simulink model "CACC_system_struct"  (Simulink 8.2)
settings: Solver=ode1  SolverMode=SingleTasking  StartTime=0.0  StopTime=inf  FixedStep=0.01  RelTol=1e-3
PreLoadFcn:
  | numd_dvsp = [0.3579 0 -0.3579];
  | dend_dvsp = [1 -1.846 0.8535];
  | simpleacc_param
PostLoadFcn:
  | , if any(exist('dsrtsu_mdlpostloadfcn', 'file') == [2, 3, 6]), try dsrtsu_mdlpostloadfcn('Execute', bdroot); catch fprintf('Error in PostLoadFcn (dsrtsu_mdlpostloadfcn) for model "%s":\n %s\n', bdroot, lasterr); end, end,
undefined symbols (not defined in the file or in its folder): command_mode, max_accel_m_s2, override_enabled, speed_command_m_s, wrench_effort_command
libraries: carma_platform x3, dsrc_transmitter x2, rtitttasklib x2, lightbar x2, srx_platform x1
(part 1 of 4)
CloseFcn:
  | rtwprivate ssgencode ModelCloseRequest Y50_MABX
settings Model: DSRTSU_INTERNAL_RTI_VER=440  DSRTSU_INTERNAL_RTI_TYPE=rti1401  DSRTSU_INTERNAL_RTIFPGA=30  Creator=N182971  LastModifiedBy=Admin  ExtModeArmWhenConnect=off  BufferReuse=off
settings DataIOCC: LimitDataPoints=off
settings OptimizationCC: BlockReduction=off  BooleanDataType=off  OptimizeBlockIOStorage=off  BufferReuse=off  ExpressionFolding=off  ExpressionDepthLimit=128  FoldNonRolledExpr=off  LocalBlockOutputs=off  InitFltsAndDblsToZero=on
settings DebuggingCC: SaveWithParameterizedLinksMsg=none  SignalResolutionControl=TryResolveAllWithWarning  SolverPrmCheckMsg=none  MultiTaskDSMMsg=warning  MultiTaskCondExecSysMsg=none  StateNameClashWarn=none
settings HardwareCC: ProdIntDivRoundTo=Zero  ProdEndianess=BigEndian  ProdHWDeviceType=Generic->Custom  TargetIntDivRoundTo=Zero  TargetEndianess=BigEndian  TargetHWDeviceType=Generic->Custom
settings RTWCC: SystemTargetFile=rti1401.tlc  MakeCommand=make_rti  TemplateMakefile=rti1401.tmf  Description=dSPACE DS1401 Hardware Platform  RTWVerbose=off  RetainRTWFile=on  ProcessScript=rti1401_make_rtw_hook  CustomSource=command_accel_encode.c  IncludeERTFirstTime=on
settings CodeAppCC: IncHierarchyInIds=on  CustomSymbolStrField=$H$N$M  CustomSymbolStrFcn=$R$H$N$M$F
settings STFCustomTargetCC: TargetFcnLib=ansi_tfl_tmw.mat  CodeReplacementLibrary=ANSI_C  ParMdlRefBuildCompliant=on  GeneratePreprocessorConditionals=Disable all  SystemTargetFile=rti1401.tlc
settings GRTTargetCC: TargetFcnLib=ansi_tfl_tmw.mat  CompOptLevelCompliant=off  ConcurrentExecutionCompliant=off  MatFileLogging=off  ExtModeMexFile=noextcomm
settings CustomProperty: DataType=RTWOptions_EnumType_C__Program Files_dSPACE RCPHIL 2014-A_MATLAB_RTI_RTI1401_TLC_rti1401_1InitialSimState  Value=RUN
settings EnumStrPairs: String=RUN

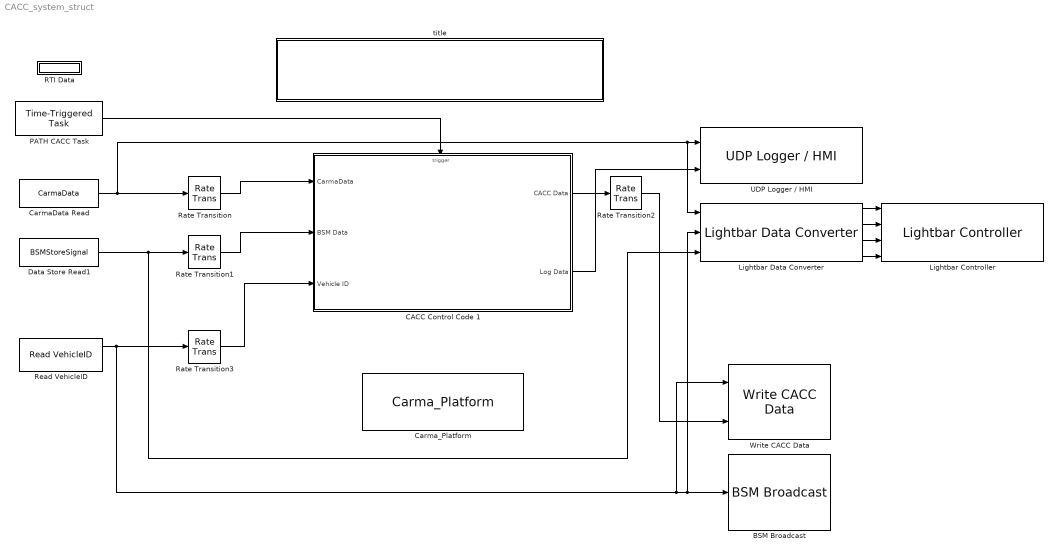
== system CACC_system_struct ==
  BSM Broadcast : dsrc_transmitter/BSM Broadcast
  CACC Control Code 1 : Subsystem
  CarmaData Read : DataStoreRead  DataStoreName=CarmaData  SampleTime=0.01  DataStoreElements=CarmaData
  "Carma_Platform " : carma_platform/Carma_Platform 
  Data Store Read1 : DataStoreRead  DataStoreName=BSMStoreSignal  SampleTime=0.01  DataStoreElements=BSMStoreSignal
  Lightbar Controller : lightbar/Lightbar Controller
  Lightbar Data Converter : lightbar/Lightbar Data Converter
  PATH CACC Task : rtitttasklib/Time-Triggered Task  TimeTriggerId=PATH_CACC  TLCFileName=rtitimetriggeredtask  DSProperties=struct('RTI',struct('Version',uint32(1),'BlockType',struct('isSLSource',uint8(1),'isSLSink',uint8(0),'isHWSource',uint8(0),'isHWSink',uint8(0),'isSetup',uint8(0),'isInline',uint8(1),'isNonInline',uint8(0),'isInterrupt',uint8(0),'isChannelwise',uint8(0)),'IOBoardType','RTITIMETRIGGER','UnitType','TIMETRIGGERED','Identifier','TASK','DialogType','SL','BlockSet','NONE','SlaveProcessor','NONE'))  RTIBlockInterface=struct('OutputPortsActive',1,'OutputPortsWidth',int32(1),'FunctionCall',uint32(0),'OutputPortsName',{{[' ']}},'InitLevel',3,'BlockDisplay',{{['Time-Triggered Task\nID: ''''PATH_CACC'''''],'center'}},'IconTransparency','off','BlockName',struct('Token',{{['Time-Triggered Task']}}),'MaskDescription',['Specifies a time-triggered task. The task trigger times are set by the assigned Time-Trigger Set block.' char(10) '' char(10) 'This block can only be used together with the Time-Trigger Set block.'])  RTIBlockParameters=struct('TimeTriggerId',{{'PATH_CACC','OFF',[]}},'TLCFileName',{{'rtitimetriggeredtask','OFF',[]}})  RTISFcnParameters=struct('TLCFileName','char')  RTIBlockParaDefault=struct('TimeTriggerId','TT_ID','TLCFileName','rtitimetriggeredtask')
  RTI Data : Subsystem  Tag=struct('RTIDataServer',struct('RTIDataServerVs','2','RTIModelDescription','struct(''main'',''CACC_system_struct'',''sub'','''',''isMp'',0)'))  LoadFcn="if exist('rtidc'), try,  rtidc('DataHostBlockClbLoad', gcbh); catch, disp(['Warning: ''LoadFcn'' for RTI Data block failed: ' lasterr]); end, end,"  mask(RTI_DATA_HOST){}
      mask help:
      | RTI Data Block.
      | This block is used by RTI to store internal model-dependent data.
      | Please keep this block on the root level of the model. Deleting this block will result in data loss.
      |
      | NEVER DELETE OR COPY THIS BLOCK!
      settings: CopyFcn="if exist('rtidc'), try,  rtidc('DataHostBlockClbCopy', gcbh); catch, disp(['Warning: ''CopyFcn'' for RTI Data block failed: ' lasterr]); end, end,"  DeleteFcn="if exist('rtidc'), try,  rtidc('DataHostBlockClbDelete', gcbh); catch, disp(['Warning: ''DeleteFcn'' for RTI Data block failed: ' lasterr]); end, end,"  ModelCloseFcn="if exist('rtidc'), try,  rtidc('DataHostBlockClbModelClose', gcbh); catch, disp(['Warning: ''ModelCloseFcn'' for RTI Data block failed: ' lasterr]); end, end,"  PreSaveFcn="if exist('rtidc'), try,  rtidc('DataHostBlockClbPreSave', gcbh); catch, disp(['Warning: ''PreSaveFcn'' for RTI Data block failed: ' lasterr]); end, end,"  PostSaveFcn="if exist('rtidc'), try,  rtidc('DataHostBlockClbPostSave', gcbh); catch, disp(['Warning: ''PostSaveFcn'' for RTI Data block failed: ' lasterr]); end, end,"  NameChangeFcn="if exist('rtidc'), try,  rtidc('DataHostBlockClbNameChange', gcbh); catch, disp(['Warning: ''NameChangeFcn'' for RTI Data block failed: ' lasterr]); end, end,"
      mask Help:
      | RTI Data Block.
      | This block is used by RTI to store internal model-dependent data.
      | Please keep this block on the root level of the model. Deleting this block will result in data loss.
      | 
      | NEVER DELETE OR COPY THIS BLOCK!
      mask Display:
      | text(0.5, 0.5, 'RTI Data', 'HorizontalAlignment', 'center');
      | plot([1 0]);
  Rate Transition{,1..3} (4 alike) : RateTransition  Deterministic=off
  Read VehicleID : srx_platform/Read VehicleID
  UDP Logger / HMI : carma_platform/UDP Logger // HMI  Value=0.05
  Write CACC Data : dsrc_transmitter/Write CACC Data
  title : Subsystem
      mask Display: disp('CACC Simulink Model')
  wires:
  PATH CACC Task/1 -> CACC Control Code 1/Trigger
  Rate Transition/1 -> CACC Control Code 1/1(CarmaData)
  CarmaData Read/1 -> Lightbar Data Converter/1, UDP Logger / HMI/1, Rate Transition/1
  Data Store Read1/1 -> Lightbar Data Converter/3, Rate Transition1/1
  Rate Transition1/1 -> CACC Control Code 1/2(BSM Data)
  Read VehicleID/1 -> Write CACC Data/1, Lightbar Data Converter/2, BSM Broadcast/1, Rate Transition3/1
  Rate Transition2/1 -> Write CACC Data/2
  Rate Transition3/1 -> CACC Control Code 1/3(Vehicle ID)
  CACC Control Code 1/1(CACC Data) -> Rate Transition2/1
  CACC Control Code 1/2(Log Data) -> UDP Logger / HMI/2
  Lightbar Data Converter/1 -> Lightbar Controller/1
  Lightbar Data Converter/2 -> Lightbar Controller/2
  Lightbar Data Converter/3 -> Lightbar Controller/3
  Lightbar Data Converter/4 -> Lightbar Controller/4

== system CACC_system_struct/CACC Control Code 1 ==
  CarmaData : Inport
  BSM Data : Inport  Port=2
  Vehicle ID : Inport  Port=3
  Trigger : TriggerPort  TriggerType=function-call  PortDimensions=1
  CAN3 TX : Subsystem
      mask Display: disp('CAN3 TX to Lower Level Control & Data Logger')
  Cadillac CACC : Subsystem
      mask Display: disp('CACC Control')
  Constant : Constant  Value=0.05
  Coordination : Subsystem
      mask Display: disp('PATH  Pos  Syst')
  Ethernet TX - to DSRC : Subsystem
      mask Display: disp('DSRC OBE TX')
  Terminator : Terminator
  Terminator1 : Terminator
  Time-Trigger Set : rtitttasklib/Time-Trigger Set  TimeTriggerId=PATH_CACC  SampleTime=-1  RegisterAtSimulationStart=on  TLCFileName=rtitimetriggerset  DSProperties=struct('RTI',struct('Version',uint32(1),'BlockType',struct('isSLSource',uint8(1),'isSLSink',uint8(0),'isHWSource',uint8(0),'isHWSink',uint8(0),'isSetup',uint8(0),'isInline',uint8(1),'isNonInline',uint8(0),'isInterrupt',uint8(0),'isChannelwise',uint8(0)),'IOBoardType','RTITIMETRIGGER','UnitType','TIMETRIGGERED','Identifier','SET','DialogType','SL','BlockSet','NONE','SlaveProcessor','NONE'))  RTIBlockInterface=struct('InputPortsActive',1,'InputPortsWidth',{{'DYNAMICALLY_SIZED'}},'InputPortsDataType',{{'SS_DOUBLE'}},'InputPortsName',{{['Trigger delay']}},'InitLevel',3,'BlockDisplay',{{['Time-Trigger Set\nID: ''''PATH_CACC'''''],'center'}},'IconTransparency','on','BlockName',struct('Token',{{['Time-Trigger Set']}}),'MaskDescription',['When this block is evaluated it sets the task trigger times for the assigned time-triggered task.' char(10) '' char(10) 'This block can only be used together with the Time-Triggered Task block.'],'SampleTime',{{-1}})  RTIBlockParameters=struct('TimeTriggerId',{{'PATH_CACC','OFF',[]}},'SampleTime',{{-1,'OFF',[]}},'RegisterAtSimulationStart',{{logical(1),'OFF',[]}},'TLCFileName',{{'rtitimetriggerset','OFF',[]}})  RTISFcnParameters=struct('TimeTriggerId','char','SampleTime','double','TLCFileName','char','RegisterAtSimulationStart','double')  RTIBlockParaDefault=struct('TimeTriggerId','TT_ID','SampleTime',-1,'RegisterAtSimulationStart',0,'TLCFileName','rtitimetriggerset')
  CACC Data : Outport
  Log Data : Outport  Port=2
  wires:
  Constant/1 -> Time-Trigger Set/1
  CarmaData/1 -> Coordination/1(CarmaData)
  BSM Data/1 -> Coordination/2(In1)
  Vehicle ID/1 -> Coordination/3(In2)
  Ethernet TX - to DSRC/1(CACC Data) -> CACC Data/1
  Cadillac CACC/1(Out1) -> Terminator/1
  Cadillac CACC/2(Out2) -> Terminator1/1
  CAN3 TX/1(Log Data) -> Log Data/1

== system CACC_system_struct/RTI Data ==
  RTI Data Store : Subsystem  Tag="struct('public',struct('sub',struct('name',{{'CACC_system_struct'}},'data',{{struct('TH',struct('thTaskInfo',struct('taskType',{'TIMER','HWINT','TMRINT','SWINT','GLINT'},'tasksNumOf',{1,1,3,0,0},'srcIds',{{'TIMERA'},{'BB_BYP_ETHT1M0I0S0'},{'INTERVALA1','INTERVALA2','INTERVALA3'},{},{}},'taskNames',{{['Timer Task 1']},{['rti_ethernet_interface_name Interrupt [RX/TX]']},{['BSM Broadcast Task'],['PATH CACC Task'],['test trigger']},{},{}})),'th_tc',struct('dataType',{'TASK','TASK','TASK','TASK','TASK'},'taskGroupId',{'','','','',''},'taskGroupList',{{},{},{},{},{}},'taskSchedulingPolicy',{'FCFS','FCFS','FCFS','FCFS','FCFS'},'taskType',{'TIMER','HWINT','TMRINT','TMRINT','TMRINT'},'blkh',{-1,['CACC_system_struct/Carma_Platform' char(10) '/SRX Platform Initializer/SRX UDP Initializer/ETHERNET_UDP_SETUP_BL1/Common Hardware' char(10) 'Interrupt Interface'],['CACC_system_struct/BSM Broadcast/BSM Broadcast Task/Common Timer' char(10) 'Interrupt Interface'],['CACC_system_struct/PATH CACC Task/Common Timer' char(10) 'Interrupt Interface'],['CACC_system_struct/UDP Logger // HMI/test trigger/Common Timer' char(10) 'Interrupt Interface']},'srcId',{'TIMERA','BB_BYP_ETHT1M0I0S0','INTERVALA1','INTERVALA2','INTERVALA3'},'srcSgnName',{['Timer A interrupt'],['BB_BYP_ETH Type 1 Module 1 HW-Int 0 Interrupt 0'],['Interval Timer A'],['Interval Timer A'],['Interval Timer A']},'srcCpuName',{'','','','',''},'taskName',{['Timer Task 1  [0.01] s'],['rti_ethernet_interface_name Interrupt [RX/TX]'],['BSM Broadcast Task'],['PATH CACC Task'],['test trigger']},'taskNameDisplayExt',{'','','','',''},'smplTime',{0.01,0,0,0,0},'smplTimeOffs',{0,0,0,0,0},'hasFixedPriority',{0,0,0,0,0},'priority',{3,2,1,4,5},'hasFixedOvc',{0,0,0,0,0},'ovcType',{1,1,1,1,1},'ovcMax',{1,1,1,1,1}),'tc_th',struct('dataType',{'TASK','TASK','TASK','TASK','TASK'},'taskGroupId',{'','','','',''},'taskGroupList',{{},{},{},{},{}},'taskSchedulingPolicy',{'FCFS','FCFS','FCFS','FCFS','FCFS'},'taskType',{'TIMER','HWINT','TMRINT','TMRINT','TMRINT'},'blkh',{-1,['CACC_system_struct/Carma_Platform' char(10) '/SRX Platform Initializer/SRX UDP Initializer/ETHERNET_UDP_SETUP_BL1/Common Hardware' char(10) 'Interrupt Interface'],['CACC_system_struct/BSM Broadcast/BSM Broadcast Task/Common Timer' char(10) 'Interrupt Interface'],['CACC_system_struct/PATH CACC Task/Common Timer' char(10) 'Interrupt Interface'],['CACC_system_struct/UDP Logger // HMI/test trigger/Common Timer' char(10) 'Interrupt Interface']},'srcId',{'TIMERA','BB_BYP_ETHT1M0I0S0','INTERVALA1','INTERVALA2','INTERVALA3'},'srcSgnName',{['Timer A interrupt'],['BB_BYP_ETH Type 1 Module 1 HW-Int 0 Interrupt 0'],['Interval Timer A'],['Interval Timer A'],['Interval Timer A']},'srcCpuName',{'','','','',''},'taskName',{['Timer Task 1  [0.01] s'],['rti_ethernet_interface_name Interrupt [RX/TX]'],['BSM Broadcast Task'],['PATH CACC Task'],['test trigger']},'taskNameDisplayExt',{'','','','',''},'smplTime',{0.01,0,0,0,0},'smplTimeOffs',{0,0,0,0,0},'hasFixedPriority',{0,0,0,0,0},'priority',{4,2,3,1,5},'hasFixedOvc',{0,0,0,0,0},'ovcType',{1,1,1,1,1},'ovcMax',{1,1,1,1,1}))}})),'private',struct('version',struct('dsVer',uint32(2)),'access',struct('modified',['09-Sep-2015 12:36:40'],'type','Model','isPerm',1)))"  mask(RTI_DATA_STORE){}
      mask help:
      | RTI Data Store Block. This block is used by RTI to store internal model dependent data. Deleting this block will result in data loss.
      |
      | NEVER DELETE, COPY, OR MODIFY THIS BLOCK!
      mask Help:
      | RTI Data Store Block. This block is used by RTI to store internal model dependent data. Deleting this block will result in data loss.
      | 
      | NEVER DELETE, COPY, OR MODIFY THIS BLOCK!
      mask Display: text(0.5, 0.5, ' ', 'HorizontalAlignment', 'center');

== system CACC_system_struct/title ==
  Constant3 : Constant  Value=0
  tag scope: Th=global, Th_1=global, hazard_h=global, trip=global, turn_sig_h=global
  wires:
  Constant3/1 -> [turn_sig_h], [Th_1], [Th], [hazard_h], [trip]

== system CACC_system_struct/CACC Control Code 1/CAN3 TX ==
  Constant : Constant
  Constant1 : Constant  Value=0
  Constant3 : Constant  Value=2
  Control Input : carma_platform/Control Input
  Get Accel Command1 : Subsystem
  Pos_&_Cotrol_to_Data_Logger : Subsystem
  Product : Product
  Switch : Switch  Threshold=1
  Terminator6 : Terminator
  Log Data : Outport
  tag scope: Control_Cmd_mode=global, Control_Overwrite_Flag=global
  wires:
  Constant/1 -> Switch/1
  Constant1/1 -> Switch/3
  Product/1 -> Switch/2
  [acc_status] -> Product/1
  [PATH_ctrl_status] -> Product/2
  Constant3/1 -> [Control_Cmd_mode]
  Switch/1 -> [Control_Overwrite_Flag]
  Get Accel Command1/1(Out1) -> Control Input/1
  Control Input/1 -> Terminator6/1
  Pos_&_Cotrol_to_Data_Logger/1(Out1) -> Log Data/1

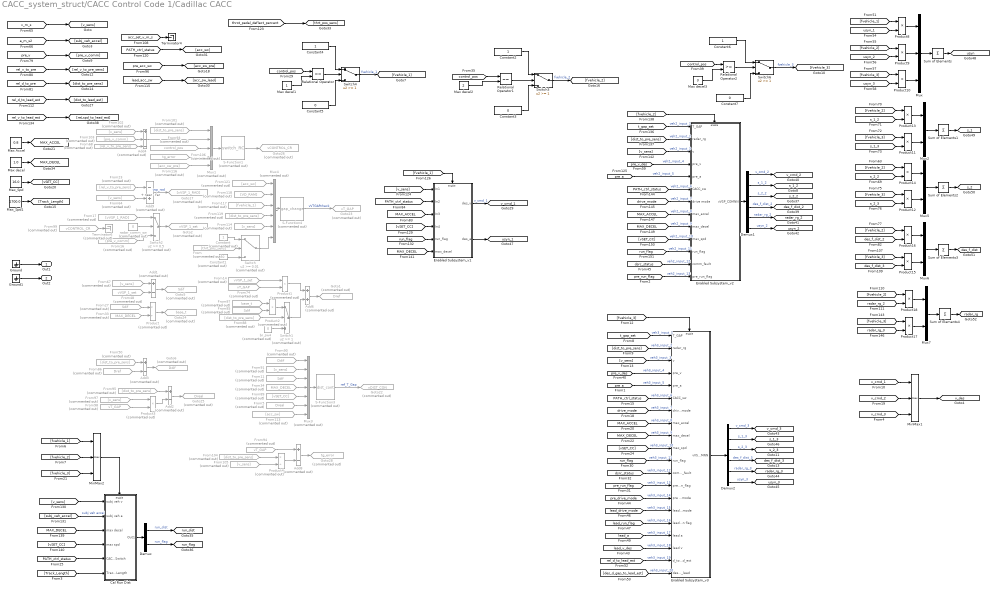
== system CACC_system_struct/CACC Control Code 1/Cadillac CACC ==
  note: + near
      | - far
  Add{1..3,8} (4 alike) : Sum  Commented=on  Inputs=+-
  Add4 : Sum  Commented=on  Inputs=+--
  Add6 : Sum  Commented=on
  Add9 : Sum  Commented=on  Inputs=-+
  Cal Run Dist : Subsystem  TreatAsAtomicUnit=on
  Constant : Constant  Commented=on
  Constant1 : Constant  Commented=on  Value=0
  Constant2 : Constant
  Constant3 : Constant  Value=0
  Constant4 : Constant
  Constant5 : Constant  Value=0
  Constant6 : Constant
  Constant7 : Constant  Value=0
  Demux : Demux  Outputs=2
  Demux1 : Demux  Outputs=6
  Demux2 : Demux  Outputs=6
  Enabled Subsystem_v1 : Subsystem  TreatAsAtomicUnit=on
  Enabled Subsystem_v2 : Subsystem  TreatAsAtomicUnit=on
  Enabled Subsystem_v3 : Subsystem  TreatAsAtomicUnit=on
  From : From  Commented=on  GotoTag=thrt_pos_sens
  From{50,88,95,101,104,119} (6 alike) : From  Commented=on  GotoTag=dist_to_pre_sens
      settings: CloseFcn=tagdialog Close
  From{64,67,91,97,102,105,114} (7 alike) : From  Commented=on  GotoTag=v_sens
      settings: CloseFcn=tagdialog Close
  From103 : From  Commented=on  GotoTag=pre_v_comm
      settings: CloseFcn=tagdialog Close
  From106 : From  Commented=on  GotoTag=tg_error  TagVisibility=global
      settings: CloseFcn=tagdialog Close
  From11 : From  Commented=on  GotoTag=Sdif  TagVisibility=global
      settings: CloseFcn=tagdialog Close
  From113 : From  Commented=on  GotoTag=acc_sw
      settings: CloseFcn=tagdialog Close
  From116 : From  Commented=on  GotoTag=acc_sw_pre
      settings: CloseFcn=tagdialog Close
  From117 : From  Commented=on  GotoTag=fvehicle_1
      settings: CloseFcn=tagdialog Close
  From118 : From  Commented=on  GotoTag=VD_RAM
      settings: CloseFcn=tagdialog Close
  From121 : From  Commented=on  GotoTag=acc_sw
      settings: CloseFcn=tagdialog Close
  From14 : From  Commented=on  GotoTag=vVSP_1_set  TagVisibility=global
      settings: CloseFcn=tagdialog Close
  From16 : From  Commented=on  GotoTag=pre_v_comm
      settings: CloseFcn=tagdialog Close
  From17 : From  Commented=on  GotoTag=vVSP_1_RAD
      settings: CloseFcn=tagdialog Close
  From23 : From  Commented=on  GotoTag=rel_v_to_pre_sens
      settings: CloseFcn=tagdialog Close
  From27 : From  Commented=on  GotoTag=Sdif  TagVisibility=global
      settings: CloseFcn=tagdialog Close
  From33 : From  Commented=on  GotoTag=MAX_DECEL  TagVisibility=global
      settings: CloseFcn=tagdialog Close
  From34 : From  Commented=on  GotoTag=MAX_DECEL  TagVisibility=global
      settings: CloseFcn=tagdialog Close
  From48 : From  Commented=on  GotoTag=vVSP_1_set  TagVisibility=global
      settings: CloseFcn=tagdialog Close
  From5 : From  Commented=on  GotoTag=Dreal  TagVisibility=global
      settings: CloseFcn=tagdialog Close
  From68 : From  Commented=on  GotoTag=rel_v_to_pre_sens
      settings: CloseFcn=tagdialog Close
  From74 : From  Commented=on  GotoTag=vT_GAP  TagVisibility=global
      settings: CloseFcn=tagdialog Close
  From85 : From  Commented=on  GotoTag=Sdif  TagVisibility=global
      settings: CloseFcn=tagdialog Close
  From86 : From  Commented=on  GotoTag=Dref  TagVisibility=global
      settings: CloseFcn=tagdialog Close
  From87 : From  Commented=on  GotoTag=base_t  TagVisibility=global
      settings: CloseFcn=tagdialog Close
  From89 : From  Commented=on  GotoTag=vSET_CC
      settings: CloseFcn=tagdialog Close
  From90 : From  Commented=on  GotoTag=Ddif  TagVisibility=global
      settings: CloseFcn=tagdialog Close
  From93 : From  Commented=on  GotoTag=control_pos  TagVisibility=global
      settings: CloseFcn=tagdialog Close
  From94 : From  Commented=on  GotoTag=vT_GAP  TagVisibility=global
      settings: CloseFcn=tagdialog Close
  From98 : From  Commented=on  GotoTag=vT_GAP  TagVisibility=global
      settings: CloseFcn=tagdialog Close
  From99 : From  Commented=on  GotoTag=vCONTROL_CR  TagVisibility=global
      settings: CloseFcn=tagdialog Close
  Goto1 : Goto  Commented=on  GotoTag=Dref  TagVisibility=global
  Goto17 : Goto  Commented=on  GotoTag=vVSP_1_RAD
  Goto2 : Goto  Commented=on  GotoTag=vVSP_1_set  TagVisibility=global
  Goto22 : Goto  Commented=on  GotoTag=vDIST_CON  TagVisibility=global
  Goto23 : Goto  Commented=on  GotoTag=vT_GAP  TagVisibility=global
  Goto24 : Goto  Commented=on  GotoTag=base_t  TagVisibility=global
  Goto25 : Goto  Commented=on  GotoTag=Dreal  TagVisibility=global
  Goto26 : Goto  Commented=on  GotoTag=vCONTROL_CR  TagVisibility=global
  Goto28 : Goto  Commented=on  GotoTag=tg_error  TagVisibility=global
  Goto5 : Goto  Commented=on  GotoTag=Sdif  TagVisibility=global
  Goto6 : Goto  Commented=on  GotoTag=Ddif  TagVisibility=global
  Ground : Ground
  Ground1 : Ground
  Max Accel : Constant  Value=0.8
  Max decel : Constant  Value=1.0
  Max decel1 : Constant
  Max decel2 : Constant  Value=2
  Max decel3 : Constant  Value=3
  Max_Spd : Constant  Value=16.0
  Max_Spd1 : Constant  Value=1700.0
  MinMax1 : MinMax  Function=max  Inputs=3
  MinMax2 : MinMax  Function=max  Inputs=3
  Mux : Mux  Inputs=3
  Mux1 : Mux  Commented=on  Inputs=5
  Mux{2,5..7} (4 alike) : Mux  Inputs=2
  Mux3 : Mux  Commented=on  Inputs=7
  Mux4 : Mux  Commented=on  Inputs=6
  Product : Product  Commented=on  Inputs=*/  RndMeth=Zero
  Product1 : Product  Commented=on  RndMeth=Zero
  Product{8..18} (11 alike) : Product
  Product2 : Product  Commented=on  RndMeth=Zero
  Product3 : Product  Commented=on  RndMeth=Zero
  Product4 : Product  Commented=on  Inputs=*/  RndMeth=Zero
  Relational Operator : RelationalOperator  Operator===  OutDataTypeStr=boolean
  Relational Operator1 : RelationalOperator  Operator===  OutDataTypeStr=boolean
  Relational Operator2 : RelationalOperator  OutDataTypeStr=boolean
  S-Function1 : S-Function  Commented=on  FunctionName=switch_RC  EnableBusSupport=off
  S-Function3 : S-Function  Commented=on  FunctionName=dist_cont  EnableBusSupport=off
  S-Function4 : S-Function  Commented=on  FunctionName=gap_change  EnableBusSupport=off
  Sum of Elements{,1..4} (5 alike) : Sum  Inputs=+
  Switch : Switch  Commented=on  Threshold=0.01
  Switch1 : Switch  Commented=on  Threshold=1  SaturateOnIntegerOverflow=on  InputSameDT=on
  Switch2 : Switch  Commented=on  Threshold=0.5  SaturateOnIntegerOverflow=on  InputSameDT=on
  Switch3 : Switch  Threshold=1
  Switch4 : Switch  Threshold=1
  Switch6 : Switch  Threshold=1
  Terminator4 : Terminator
  Terminator6 : Terminator  Commented=on
  br_sw4 : Constant  Commented=on  Value=0
  radar_comm_sw : Constant  Commented=on  Value=0
  Out1 : Outport
  Out2 : Outport  Port=2
  tag scope: MAX_ACCEL=global, MAX_DECEL=global, des_f_dist=global, des_f_dist_2=global, des_f_dist_3=global, radar_rg=global, radar_rg_2=global, radar_rg_3=global, run_dist=global, run_flag=global, s_1=global, s_1_2=global, s_1_3=global, s_2=global, s_2_2=global, s_2_3=global, usyn=global, usyn_1=global, usyn_2=global, usyn_3=global, v_cmd_1=global, v_cmd_2=global, v_cmd_3=global, v_des=global
  wires:
  Ground/1 -> Out1/1
  Ground1/1 -> Out2/1
  Max Accel/1 -> [MAX_ACCEL]
  Mux1/1 -> S-Function1/1
  S-Function1/1 -> Goto26/1
  From102/1 -> Add4/1
  From103/1 -> Add4/2
  From68/1 -> Add4/3
  Add4/1 -> Mux1/2
  From101/1 -> Mux1/1
  From93/1 -> Mux1/3
  From106/1 -> Mux1/4
  From116/1 -> Mux1/5
  From17/1 -> Switch2/1
  From16/1 -> Switch2/3
  From50/1 -> Add3/1
  From86/1 -> Add3/2
  Add3/1 -> Goto6/1
  Mux3/1 -> S-Function3/1
  S-Function3/1 -> Goto22/1  "ref_T_Gap"
  From90/1 -> Mux3/1
  From91/1 -> Mux3/2
  From67/1 -> Add1/1
  From48/1 -> Add1/2
  Add1/1 -> Goto5/1
  From11/1 -> Mux3/3
  From34/1 -> Mux3/4
  From95/1 -> Add2/1
  Product3/1 -> Add2/2
  From97/1 -> Product3/1
  From98/1 -> Product3/2
  Add2/1 -> Goto25/1
  From5/1 -> Mux3/6
  From27/1 -> Product/1
  From33/1 -> Product/2
  Product/1 -> Goto24/1
  From87/1 -> Product2/1
  From74/1 -> Product1/2
  From14/1 -> Product1/1
  From85/1 -> Product2/2
  Product1/1 -> Add6/1
  Add6/1 -> Goto1/1
  Product2/1 -> Switch1/1
  br_sw4/1 -> Switch1/3
  From88/1 -> Switch1/2
  Switch1/1 -> Add6/2
  From89/1 -> Mux3/5
  From105/1 -> Product4/2
  From104/1 -> Product4/1
  From94/1 -> Add8/1
  Product4/1 -> Add8/2
  Add8/1 -> Goto28/1
  From113/1 -> Mux3/7
  Switch2/1 -> Goto2/1
  Mux4/1 -> S-Function4/1
  From121/1 -> Mux4/1
  From118/1 -> Mux4/2
  From117/1 -> Mux4/3
  From119/1 -> Mux4/4
  Switch/1 -> Mux4/6
  From114/1 -> Mux4/5
  S-Function4/1 -> Goto23/1  "vVTGAPcheck"
  [v_cmd_2] -> MinMax1/2
  [v_cmd_3] -> MinMax1/3
  MinMax1/1 -> [v_des]
  Add9/1 -> Goto17/1  "vsp_rad"
  From64/1 -> Add9/2
  From23/1 -> Add9/1
  Constant/1 -> Switch/1
  Constant1/1 -> Switch/3
  From/1 -> Switch/2
  [v_m_s] -> [v_sens]
  [a_m_s2] -> [subj_veh_accel]
  [pre_v] -> [pre_v_comm]
  [rel_v_to_pre] -> [rel_v_to_pre_sens]
  [rel_d_to_pre] -> [dist_to_pre_sens]
  [acc_set_v_m_s] -> Terminator4/1
  [PATH_ctrl_status] -> [acc_sw]
  [pre_acc_sw] -> [acc_sw_pre]
  [lead_acc_sw] -> [acc_sw_lead]
  [v_cmd_1] -> MinMax1/1
  Max decel/1 -> [MAX_DECEL]
  Max_Spd/1 -> [vSET_CC]
  From99/1 -> Terminator6/1
  radar_comm_sw/1 -> Switch2/2
  [rel_d_to_lead_est] -> [dist_to_lead_est]
  [rel_v_to_lead_est] -> [reLspd_to_lead_est]
  [fvehicle_2] -> Enabled Subsystem_v2/Enable
  [t_gap_set] -> Enabled Subsystem_v2/1(T_GAP)  "veh2_input_1"
  [dist_to_pre_sens] -> Enabled Subsystem_v2/2(radar_rg)  "veh2_input_2"
  [v_sens] -> Enabled Subsystem_v2/3(v)  "veh2_input_3"
  [PATH_ctrl_status] -> Enabled Subsystem_v2/6(CACC_sw)  "veh2_input_6"
  [drive_mode] -> Enabled Subsystem_v2/7(drive mode)  "veh2_input_7"
  [MAX_ACCEL] -> Enabled Subsystem_v2/8(max_accel)  "veh2_input_8"
  [MAX_DECEL] -> Enabled Subsystem_v2/9(max_decel)  "veh2_input_9"
  [vSET_CC] -> Enabled Subsystem_v2/10(max_spd)  "veh2_input_10"
  [run_flag] -> Enabled Subsystem_v2/11(run_flag)  "veh2_input_11"
  [dsrc_status] -> Enabled Subsystem_v2/12(comm_fault)  "veh2_input_12"
  [v_sens] -> Cal Run Dist/1(subj veh v)
  [subj_veh_accel] -> Cal Run Dist/2(subj veh a)  "subj veh accel"
  Cal Run Dist/1(Out1) -> Demux/1
  Demux/1 -> [run_dist]  "run_dist"
  Demux/2 -> [run_flag]  "run_flag"
  [MAX_DECEL] -> Cal Run Dist/3(max decel)
  [vSET_CC] -> Cal Run Dist/4(max spd)
  [PATH_ctrl_status] -> Cal Run Dist/5(CACC_Switch)
  [v_sens] -> Enabled Subsystem_v1/1(In1)
  Enabled Subsystem_v1/1(des_v) -> [v_cmd_1]  "v_cmd_1"
  [fvehicle_1] -> Enabled Subsystem_v1/Enable
  [MAX_ACCEL] -> Enabled Subsystem_v1/3(In3)
  [vSET_CC] -> Enabled Subsystem_v1/4(In4)
  [PATH_ctrl_status] -> Enabled Subsystem_v1/2(In2)
  [run_flag] -> Enabled Subsystem_v1/5(run_flag)
  [MAX_DECEL] -> Enabled Subsystem_v1/6(max_decel)
  Enabled Subsystem_v2/1(vVSP_COMNN) -> Demux1/1
  Demux1/1 -> [v_cmd_2]  "v_cmd_2"
  Demux1/2 -> [s_1_2]  "s_1_2"
  Demux1/3 -> [s_2_2]  "s_2_2"
  Demux1/4 -> [des_f_dist_2]  "des_f_dist_2"
  Demux1/5 -> [radar_rg_2]  "radar_rg_2"
  Demux1/6 -> [usyn_2]  "usyn_2"
  [pre_v_des] -> Enabled Subsystem_v2/4(pre_v)  "veh2_input_4"
  [pre_a] -> Enabled Subsystem_v2/5(pre_a)  "veh2_input_5"
  [pre_run_flag] -> Enabled Subsystem_v2/13(pre_run_flag)  "veh2_input_13"
  [Track_Length] -> Cal Run Dist/6(Track_Length)
  Max_Spd1/1 -> [Track_Length]
  [fvehicle_3] -> Enabled Subsystem_v3/Enable
  [t_gap_set] -> Enabled Subsystem_v3/1(T_GAP)  "veh3_input_1"
  [dist_to_pre_sens] -> Enabled Subsystem_v3/2(radar_rg)  "veh3_input_2"
  [v_sens] -> Enabled Subsystem_v3/3(v)  "veh3_input_3"
  [PATH_ctrl_status] -> Enabled Subsystem_v3/6(CACC_sw)  "veh3_input_6"
  [drive_mode] -> Enabled Subsystem_v3/7(drive mode)  "veh3_input_7"
  [MAX_ACCEL] -> Enabled Subsystem_v3/8(max_accel)  "veh3_input_8"
  [MAX_DECEL] -> Enabled Subsystem_v3/9(max_decel)  "veh3_input_9"
  [vSET_CC] -> Enabled Subsystem_v3/10(max_spd)  "veh3_input_10"
  [run_flag] -> Enabled Subsystem_v3/11(run_flag)  "veh3_input_11"
  [dsrc_status] -> Enabled Subsystem_v3/12(comm_fault)  "veh3_input_12"
  Enabled Subsystem_v3/1(vVSP_COMNN) -> Demux2/1
  Demux2/1 -> [v_cmd_3]  "v_cmd_3"
  Demux2/2 -> [s_1_3]  "s_1_3"
  Demux2/3 -> [s_2_3]  "s_2_3"
  Demux2/4 -> [des_f_dist_3]  "des_f_dist_3"
  Demux2/5 -> [radar_rg_3]  "radar_rg_3"
  Demux2/6 -> [usyn_3]  "usyn_3"
  [pre_v_des] -> Enabled Subsystem_v3/4(pre_v)  "veh3_input_4"
  [pre_a] -> Enabled Subsystem_v3/5(pre_a)  "veh3_input_5"
  [pre_run_flag] -> Enabled Subsystem_v3/13(pre_run_flag)  "veh3_input_13"
  [pre_drive_mode] -> Enabled Subsystem_v3/14(pre drive mode)  "veh3_input_14"
  [lead_drive_mode] -> Enabled Subsystem_v3/15(lead drive mode)  "veh3_input_15"
  [lead_run_flag] -> Enabled Subsystem_v3/16(lead run flag)  "veh3_input_16"
  [lead_a] -> Enabled Subsystem_v3/17(lead a)  "veh3_input_17"
  [lead_v_des] -> Enabled Subsystem_v3/18(lead v)  "veh3_input_18"
  [rel_d_to_lead_est] -> Enabled Subsystem_v3/19(d_to_lead_est)  "veh3_input_19"
  [des_d_gap_to_lead_est] -> Enabled Subsystem_v3/20(des_d_gap_to_lead)  "veh3_input_20"
  Enabled Subsystem_v1/2(des_a) -> [usyn_1]
  Mux/1 -> Sum of Elements/1
  Product8/1 -> Mux/1
  [fvehicle_1] -> Product8/1
  [usyn_1] -> Product8/2
  Product9/1 -> Mux/2
  [fvehicle_2] -> Product9/1
  [usyn_2] -> Product9/2
  [fvehicle_3] -> Product10/1
  [usyn_3] -> Product10/2
  Product10/1 -> Mux/3
  Sum of Elements/1 -> [usyn]
  Mux2/1 -> Sum of Elements1/1
  Product13/1 -> Mux2/1
  [fvehicle_2] -> Product13/1
  [s_1_2] -> Product13/2
  [fvehicle_3] -> Product11/1
  [s_1_3] -> Product11/2
  Sum of Elements1/1 -> [s_1]
  Product11/1 -> Mux2/2
  Mux5/1 -> Sum of Elements2/1
  Product14/1 -> Mux5/1
  [fvehicle_2] -> Product14/1
  [s_2_2] -> Product14/2
  [fvehicle_3] -> Product12/1
  [s_2_3] -> Product12/2
  Sum of Elements2/1 -> [s_2]
  Product12/1 -> Mux5/2
  Mux6/1 -> Sum of Elements3/1
  Product16/1 -> Mux6/1
  [fvehicle_2] -> Product16/1
  [des_f_dist_2] -> Product16/2
  [fvehicle_3] -> Product15/1
  [des_f_dist_3] -> Product15/2
  Sum of Elements3/1 -> [des_f_dist]
  Product15/1 -> Mux6/2
  Mux7/1 -> Sum of Elements4/1
  Product18/1 -> Mux7/1
  [fvehicle_2] -> Product18/1
  [radar_rg_2] -> Product18/2
  [fvehicle_3] -> Product17/1
  [radar_rg_3] -> Product17/2
  Sum of Elements4/1 -> [radar_rg]
  Product17/1 -> Mux7/2
  Constant2/1 -> Switch3/1
  Constant3/1 -> Switch3/3
  Constant4/1 -> Switch4/1
  Constant5/1 -> Switch4/3
  Relational Operator/1 -> Switch4/2
  [control_pos] -> Relational Operator/1
  Max decel1/1 -> Relational Operator/2
  [control_pos] -> Relational Operator1/1
  Max decel2/1 -> Relational Operator1/2
  Constant7/1 -> Switch6/3
  Switch6/1 -> [fvehicle_3]  "fvehicle_3"
  [control_pos] -> Relational Operator2/1
  Max decel3/1 -> Relational Operator2/2
  Switch4/1 -> [fvehicle_1]  "fvehicle_1"
  Switch3/1 -> [fvehicle_2]  "fvehicle_2"
  Relational Operator1/1 -> Switch3/2
  Relational Operator2/1 -> Switch6/2
  Constant6/1 -> Switch6/1
  [throt_pedal_deflect_percent] -> [thrt_pos_sens]
  [fvehicle_1] -> MinMax2/1
  [fvehicle_2] -> MinMax2/2
  [fvehicle_3] -> MinMax2/3
  MinMax2/1 -> Cal Run Dist/Enable

== system CACC_system_struct/CACC Control Code 1/Coordination ==
  CarmaData : Inport
  In1 : Inport  Port=2  OutDataTypeStr=Bus: BSMStoreBus
  In2 : Inport  Port=3
  Activation : Subsystem
  BSM 1 : Subsystem
  BSM 2 : Subsystem
  BSM 3 : Subsystem
  BSM 4 : Subsystem
  BSM 5 : Subsystem
  BSM_1 : Subsystem
  BSM_2 : Subsystem
  BSM_3 : Subsystem
  BSM_4 : Subsystem
  BSM_5 : Subsystem
  Bus Selector : BusSelector  OutputSignals=Veh1BSM,Veh2BSM,Veh3BSM,Veh4BSM,Veh5BSM
  Constant : Constant  Value=2
  Coordination : S-Function  FunctionName=coordination  EnableBusSupport=off
  Data Type Conversion : DataTypeConversion
  JBus_data : Subsystem
  MATLAB Function : MATLAB Function  TreatAsAtomicUnit=on
  Mux : Mux  Inputs=16
  Subj_veh_info : Subsystem
  Veh Pos Input : Subsystem
  Veh Pos Output : Subsystem
  lead_veh : Subsystem
  pre_veh : Subsystem
  subj_veh : Subsystem
  tag scope: cacc_grp_len=global, subj_veh_id=global
  wires:
  BSM 1/1(Out1) -> Coordination/2
  Coordination/1 -> Activation/1(In1)
  BSM 4/1(Out1) -> Coordination/5
  BSM 3/1(Out1) -> Coordination/4
  MATLAB Function/1(y) -> Veh Pos Output/1(In1)
  BSM 5/1(Out1) -> Coordination/6
  BSM 2/1(Out1) -> Coordination/3
  JBus_data/1(Out1) -> Coordination/7
  Constant/1 -> [cacc_grp_len]
  Coordination/4 -> lead_veh/1(In1)
  Coordination/3 -> pre_veh/1(In1)
  Coordination/2 -> subj_veh/1(In1)
  Veh Pos Input/1(Out1) -> Coordination/1
  [local_enu_E_1] -> Mux/2
  [local_enu_N_1] -> Mux/3
  [veh_id_1] -> Mux/1
  [local_enu_E_2] -> Mux/5
  [local_enu_N_2] -> Mux/6
  [veh_id_2] -> Mux/4
  [local_enu_E_3] -> Mux/8
  [local_enu_N_3] -> Mux/9
  [veh_id_3] -> Mux/7
  [local_enu_E_4] -> Mux/11
  [local_enu_N_4] -> Mux/12
  [veh_id_4] -> Mux/10
  [local_enu_E_5] -> Mux/14
  [local_enu_N_5] -> Mux/15
  [veh_id_5] -> Mux/13
  [cacc_grp_len] -> Mux/16
  Mux/1 -> MATLAB Function/1(u)
  Subj_veh_info/1(Out1) -> Coordination/8
  CarmaData/1 -> JBus_data/1(CarmaData)
  In1/1 -> Bus Selector/1
  Bus Selector/1 -> BSM_1/1(Vehicle1 BSM)  "<Veh1BSM>"
  Bus Selector/2 -> BSM_2/1(Vehicle2 BSM)  "<Veh2BSM>"
  Bus Selector/3 -> BSM_3/1(Vehicle3 BSM)  "<Veh3BSM>"
  Bus Selector/4 -> BSM_4/1(Vehicle4 BSM)  "<Veh4BSM>"
  Bus Selector/5 -> BSM_5/1(Vehicle5 BSM)  "<Veh5BSM>"
  In2/1 -> Data Type Conversion/1
  Data Type Conversion/1 -> [subj_veh_id]

== system CACC_system_struct/CACC Control Code 1/Ethernet TX - to DSRC ==
  Subj_Veh_Msg_to_Memory_Store : Subsystem
  CACC Data : Outport
  wires:
  Subj_Veh_Msg_to_Memory_Store/1(CACC Data) -> CACC Data/1

== system CACC_system_struct/RTI Data/RTI Data Store ==
  RTI Data Store : Subsystem  mask(RTI_DATA_STORE){}
      mask help:
      | RTI Data Store Block. This block is used by RTI to store internal model dependent data. Deleting this block will result in data loss.
      |
      | NEVER DELETE, COPY, OR MODIFY THIS BLOCK!
      mask Help:
      | RTI Data Store Block. This block is used by RTI to store internal model dependent data. Deleting this block will result in data loss.
      | 
      | NEVER DELETE, COPY, OR MODIFY THIS BLOCK!
      mask Display: text(0.5, 0.5, ' ', 'HorizontalAlignment', 'center');

== system CACC_system_struct/CACC Control Code 1/CAN3 TX/Get Accel Command1 ==
  Accel Zero Command : Constant  Value=0  OutDataTypeStr=Bus: AccelCommandBus
  Bus Assignment : BusAssignment  AssignedSignals=override_enabled,command_mode,wrench_effort_command,speed_command_m_s,max_accel_m_s2
  Data Type Conversion1 : DataTypeConversion  OutDataTypeStr=Enum: AccelCommandMode
  Data Type Conversion17 : DataTypeConversion  OutDataTypeStr=boolean
  Data Type Conversion2 : DataTypeConversion  OutMin=[0]  OutMax=[5]  OutDataTypeStr=double
  Data Type Conversion3 : DataTypeConversion  OutMin=[0]  OutMax=[5]  OutDataTypeStr=double
  Data Type Conversion4 : DataTypeConversion  OutMin=[0]  OutMax=[5]  OutDataTypeStr=double
  Data Type Conversion5 : DataTypeConversion  OutDataTypeStr=uint32
  Out1 : Outport
  wires:
  [Control_Overwrite_Flag] -> Data Type Conversion17/1
  [Control_Cmd_mode] -> Data Type Conversion5/1
  [torq_des] -> Data Type Conversion2/1
  [v_des] -> Data Type Conversion3/1
  [MAX_ACCEL] -> Data Type Conversion4/1
  Data Type Conversion17/1 -> Bus Assignment/2
  Data Type Conversion1/1 -> Bus Assignment/3
  Data Type Conversion2/1 -> Bus Assignment/4
  Data Type Conversion3/1 -> Bus Assignment/5
  Data Type Conversion4/1 -> Bus Assignment/6
  Accel Zero Command/1 -> Bus Assignment/1
  Bus Assignment/1 -> Out1/1
  Data Type Conversion5/1 -> Data Type Conversion1/1

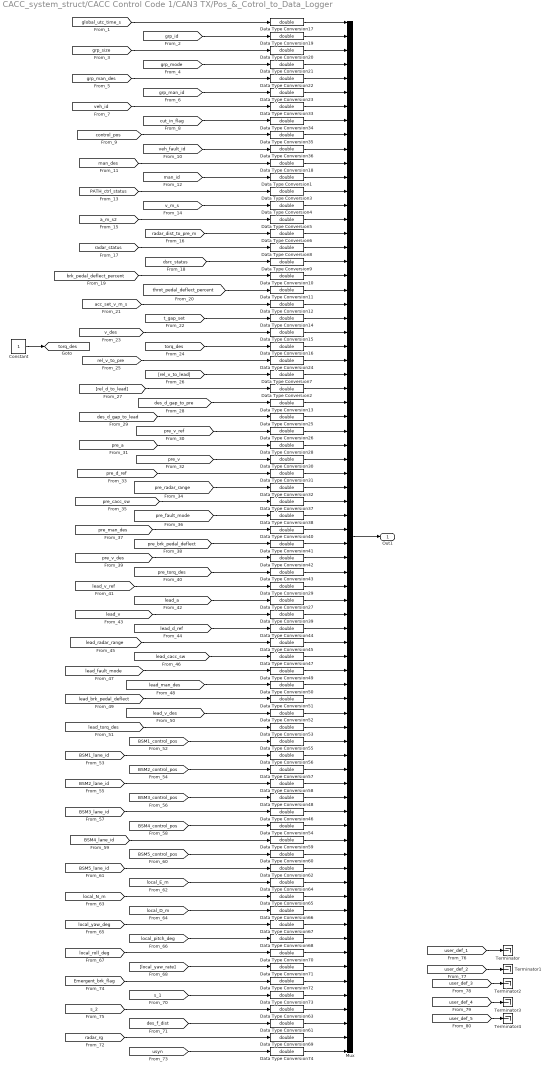
== system CACC_system_struct/CACC Control Code 1/CAN3 TX/Pos_&_Cotrol_to_Data_Logger ==
  Constant : Constant
  Data Type Conversion{1..74} (74 alike) : DataTypeConversion  OutMin=[0]  OutMax=[5]  OutDataTypeStr=double
  Mux : Mux  Inputs=74
  Terminator{,1..4} (5 alike) : Terminator
  Out1 : Outport
  tag scope: torq_des=global
  wires:
  Mux/1 -> Out1/1
  [global_utc_time_s] -> Data Type Conversion17/1
  [grp_id] -> Data Type Conversion19/1
  [grp_size] -> Data Type Conversion20/1
  [grp_mode] -> Data Type Conversion21/1
  [grp_man_des] -> Data Type Conversion22/1
  [grp_man_id] -> Data Type Conversion23/1
  [veh_id] -> Data Type Conversion33/1
  [cut_in_flag] -> Data Type Conversion34/1
  [control_pos] -> Data Type Conversion35/1
  [veh_fault_id] -> Data Type Conversion36/1
  [man_des] -> Data Type Conversion18/1
  [man_id] -> Data Type Conversion1/1
  [PATH_ctrl_status] -> Data Type Conversion3/1
  [v_m_s] -> Data Type Conversion4/1
  [a_m_s2] -> Data Type Conversion5/1
  [radar_dist_to_pre_m] -> Data Type Conversion6/1
  [dsrc_status] -> Data Type Conversion9/1
  [brk_pedal_deflect_percent] -> Data Type Conversion10/1
  [throt_pedal_deflect_percent] -> Data Type Conversion11/1
  [acc_set_v_m_s] -> Data Type Conversion12/1
  [v_des] -> Data Type Conversion15/1
  [torq_des] -> Data Type Conversion16/1
  [rel_v_to_pre] -> Data Type Conversion24/1
  [rel_v_to_lead] -> Data Type Conversion7/1
  [rel_d_to_lead] -> Data Type Conversion2/1
  [des_d_gap_to_pre] -> Data Type Conversion13/1
  [des_d_gap_to_lead] -> Data Type Conversion25/1
  [pre_v_ref] -> Data Type Conversion26/1
  [pre_a] -> Data Type Conversion28/1
  [pre_v] -> Data Type Conversion30/1
  [pre_d_ref] -> Data Type Conversion31/1
  [pre_radar_range] -> Data Type Conversion32/1
  [pre_cacc_sw] -> Data Type Conversion37/1
  [pre_fault_mode] -> Data Type Conversion38/1
  [pre_man_des] -> Data Type Conversion40/1
  [pre_brk_pedal_deflect] -> Data Type Conversion41/1
  [pre_v_des] -> Data Type Conversion42/1
  [pre_torq_des] -> Data Type Conversion43/1
  [lead_v_ref] -> Data Type Conversion29/1
  [lead_a] -> Data Type Conversion27/1
  [lead_v] -> Data Type Conversion39/1
  [lead_d_ref] -> Data Type Conversion44/1
  [lead_radar_range] -> Data Type Conversion45/1
  [lead_cacc_sw] -> Data Type Conversion47/1
  [lead_fault_mode] -> Data Type Conversion49/1
  [lead_man_des] -> Data Type Conversion50/1
  [lead_brk_pedal_deflect] -> Data Type Conversion51/1
  [lead_v_des] -> Data Type Conversion52/1
  [lead_torq_des] -> Data Type Conversion53/1
  [BSM1_control_pos] -> Data Type Conversion55/1
  [BSM1_lane_id] -> Data Type Conversion56/1
  [BSM2_control_pos] -> Data Type Conversion57/1
  [BSM2_lane_id] -> Data Type Conversion58/1
  [BSM3_control_pos] -> Data Type Conversion48/1
  [BSM3_lane_id] -> Data Type Conversion46/1
  [BSM4_control_pos] -> Data Type Conversion54/1
  [BSM4_lane_id] -> Data Type Conversion59/1
  [BSM5_control_pos] -> Data Type Conversion60/1
  [BSM5_lane_id] -> Data Type Conversion62/1
  [local_E_m] -> Data Type Conversion64/1
  [local_N_m] -> Data Type Conversion65/1
  [local_D_m] -> Data Type Conversion66/1
  [local_yaw_deg] -> Data Type Conversion67/1
  [local_pitch_deg] -> Data Type Conversion68/1
  [local_roll_deg] -> Data Type Conversion70/1
  [local_yaw_rate] -> Data Type Conversion71/1
  [t_gap_set] -> Data Type Conversion14/1
  [radar_status] -> Data Type Conversion8/1
  Data Type Conversion17/1 -> Mux/1
  Data Type Conversion19/1 -> Mux/2
  Data Type Conversion20/1 -> Mux/3
  Data Type Conversion21/1 -> Mux/4
  Data Type Conversion22/1 -> Mux/5
  Data Type Conversion23/1 -> Mux/6
  Data Type Conversion36/1 -> Mux/10
  Data Type Conversion5/1 -> Mux/15
  Data Type Conversion18/1 -> Mux/11
  Data Type Conversion33/1 -> Mux/7
  Data Type Conversion3/1 -> Mux/13
  Data Type Conversion34/1 -> Mux/8
  Data Type Conversion35/1 -> Mux/9
  Data Type Conversion1/1 -> Mux/12
  Data Type Conversion4/1 -> Mux/14
  Data Type Conversion9/1 -> Mux/18
  Data Type Conversion13/1 -> Mux/28
  Data Type Conversion25/1 -> Mux/29
  Data Type Conversion10/1 -> Mux/19
  Data Type Conversion8/1 -> Mux/17
  Data Type Conversion26/1 -> Mux/30
  Data Type Conversion7/1 -> Mux/26
  Data Type Conversion15/1 -> Mux/23
  Data Type Conversion16/1 -> Mux/24
  Data Type Conversion14/1 -> Mux/22
  Data Type Conversion2/1 -> Mux/27
  Data Type Conversion6/1 -> Mux/16
  Data Type Conversion12/1 -> Mux/21
  Data Type Conversion24/1 -> Mux/25
  Data Type Conversion11/1 -> Mux/20
  Data Type Conversion45/1 -> Mux/45
  Data Type Conversion44/1 -> Mux/44
  Data Type Conversion43/1 -> Mux/40
  Data Type Conversion42/1 -> Mux/39
  Data Type Conversion41/1 -> Mux/38
  Data Type Conversion40/1 -> Mux/37
  Data Type Conversion39/1 -> Mux/43
  Data Type Conversion38/1 -> Mux/36
  Data Type Conversion37/1 -> Mux/35
  Data Type Conversion32/1 -> Mux/34
  Data Type Conversion31/1 -> Mux/33
  Data Type Conversion30/1 -> Mux/32
  Data Type Conversion29/1 -> Mux/41
  Data Type Conversion28/1 -> Mux/31
  Data Type Conversion27/1 -> Mux/42
  Data Type Conversion46/1 -> Mux/57
  Data Type Conversion50/1 -> Mux/48
  Data Type Conversion49/1 -> Mux/47
  Data Type Conversion59/1 -> Mux/59
  Data Type Conversion51/1 -> Mux/49
  Data Type Conversion52/1 -> Mux/50
  Data Type Conversion60/1 -> Mux/60
  Data Type Conversion47/1 -> Mux/46
  Data Type Conversion53/1 -> Mux/51
  Data Type Conversion56/1 -> Mux/53
  Data Type Conversion54/1 -> Mux/58
  Data Type Conversion55/1 -> Mux/52
  Data Type Conversion58/1 -> Mux/55
  Data Type Conversion57/1 -> Mux/54
  Data Type Conversion48/1 -> Mux/56
  Data Type Conversion65/1 -> Mux/63
  Data Type Conversion73/1 -> Mux/70
  Data Type Conversion69/1 -> Mux/73
  Data Type Conversion71/1 -> Mux/68
  Data Type Conversion70/1 -> Mux/67
  Data Type Conversion62/1 -> Mux/61
  Data Type Conversion68/1 -> Mux/66
  Data Type Conversion63/1 -> Mux/71
  Data Type Conversion64/1 -> Mux/62
  Data Type Conversion67/1 -> Mux/65
  Data Type Conversion66/1 -> Mux/64
  Data Type Conversion72/1 -> Mux/69
  Data Type Conversion74/1 -> Mux/74
  Data Type Conversion61/1 -> Mux/72
  Constant/1 -> [torq_des]
  [user_def_1] -> Terminator/1
  [user_def_2] -> Terminator1/1
  [user_def_3] -> Terminator2/1
  [user_def_4] -> Terminator3/1
  [user_def_5] -> Terminator4/1
  [des_f_dist] -> Data Type Conversion61/1
  [radar_rg] -> Data Type Conversion69/1
  [Emergent_brk_flag] -> Data Type Conversion72/1
  [usyn] -> Data Type Conversion74/1
  [s_1] -> Data Type Conversion73/1
  [s_2] -> Data Type Conversion63/1

== system CACC_system_struct/CACC Control Code 1/Cadillac CACC/Cal Run Dist ==
  subj veh v : Inport
  subj veh a : Inport  Port=2
  max decel : Inport  Port=3
  max spd : Inport  Port=4
  CACC_Switch : Inport  Port=5
  Track_Length : Inport  Port=6
  Enable Run Dist : EnablePort
  Mux : Mux  Inputs=6
  S-Function2 : S-Function  FunctionName=run_dist  EnableBusSupport=off
  Out1 : Outport
  wires:
  S-Function2/1 -> Out1/1  "run_dist"
  subj veh v/1 -> Mux/1
  subj veh a/1 -> Mux/2
  Mux/1 -> S-Function2/1
  max decel/1 -> Mux/3
  max spd/1 -> Mux/4
  CACC_Switch/1 -> Mux/5
  Track_Length/1 -> Mux/6

== system CACC_system_struct/CACC Control Code 1/Cadillac CACC/Enabled Subsystem_v1 ==
  In1 : Inport
  In2 : Inport  Port=2
  In3 : Inport  Port=3
  In4 : Inport  Port=4
  run_flag : Inport  Port=5
  max_decel : Inport  Port=6
  Enable : EnablePort
  Demux : Demux  Outputs=2
  Mux : Mux  Inputs=6
  S-Function2 : S-Function  FunctionName=cc_v_ref  EnableBusSupport=off
  des_v : Outport
  des_a : Outport  Port=2
  wires:
  S-Function2/1 -> Demux/1
  In1/1 -> Mux/1
  Mux/1 -> S-Function2/1
  In2/1 -> Mux/2
  In3/1 -> Mux/3
  In4/1 -> Mux/4
  run_flag/1 -> Mux/5
  max_decel/1 -> Mux/6
  Demux/1 -> des_v/1
  Demux/2 -> des_a/1

== system CACC_system_struct/CACC Control Code 1/Cadillac CACC/Enabled Subsystem_v2 ==
  T_GAP : Inport
  radar_rg : Inport  Port=2
  v : Inport  Port=3
  pre_v : Inport  Port=4
  pre_a : Inport  Port=5
  CACC_sw : Inport  Port=6
  drive mode : Inport  Port=7
  max_accel : Inport  Port=8
  max_decel : Inport  Port=9
  max_spd : Inport  Port=10
  run_flag : Inport  Port=11
  comm_fault : Inport  Port=12
  pre_run_flag : Inport  Port=13
  Enable : EnablePort  StatesWhenEnabling=reset
  Mux : Mux  Inputs=13
  S-Func : S-Function  FunctionName=dist_contr  EnableBusSupport=off
  vVSP_COMNN : Outport  OutputWhenDisabled=reset  InitialOutput=0
  wires:
  S-Func/1 -> vVSP_COMNN/1
  Mux/1 -> S-Func/1  "speed_command"
  T_GAP/1 -> Mux/1  "veh2_t_GAP"
  radar_rg/1 -> Mux/2  "veh2_radar_range"
  v/1 -> Mux/3  "veh2_v"
  pre_v/1 -> Mux/4  "veh2_pre_v"
  pre_a/1 -> Mux/5  "veh2_pre_a"
  CACC_sw/1 -> Mux/6  "veh2_CACC_sw"
  drive mode/1 -> Mux/7  "veh2_drive_mode"
  max_accel/1 -> Mux/8  "veh2_max_accel"
  max_decel/1 -> Mux/9  "veh2_max_decel"
  max_spd/1 -> Mux/10  "veh2_max_spd"
  run_flag/1 -> Mux/11  "veh2_run_flag"
  comm_fault/1 -> Mux/12  "comm_pre_fault"
  pre_run_flag/1 -> Mux/13  "pre_run_flag"

== system CACC_system_struct/CACC Control Code 1/Cadillac CACC/Enabled Subsystem_v3 ==
  T_GAP : Inport
  radar_rg : Inport  Port=2
  v : Inport  Port=3
  pre_v : Inport  Port=4
  pre_a : Inport  Port=5
  CACC_sw : Inport  Port=6
  drive mode : Inport  Port=7
  max_accel : Inport  Port=8
  max_decel : Inport  Port=9
  max_spd : Inport  Port=10
  run_flag : Inport  Port=11
  comm_fault : Inport  Port=12
  pre_run_flag : Inport  Port=13
  pre drive mode : Inport  Port=14
  lead drive mode : Inport  Port=15
  lead run flag : Inport  Port=16
  lead a : Inport  Port=17
  lead v : Inport  Port=18
  d_to_lead_est : Inport  Port=19
  des_d_gap_to_lead : Inport  Port=20
  Enable : EnablePort  StatesWhenEnabling=reset
  Mux : Mux  Inputs=20
  S-Func : S-Function  FunctionName=dist_contr_n  EnableBusSupport=off
  vVSP_COMNN : Outport  OutputWhenDisabled=reset  InitialOutput=0
  wires:
  S-Func/1 -> vVSP_COMNN/1
  Mux/1 -> S-Func/1
  T_GAP/1 -> Mux/1  "veh2_t_GAP"
  radar_rg/1 -> Mux/2  "veh2_radar_range"
  v/1 -> Mux/3  "veh2_v"
  pre_v/1 -> Mux/4  "veh2_pre_v"
  pre_a/1 -> Mux/5  "veh2_pre_a"
  CACC_sw/1 -> Mux/6  "veh2_CACC_sw"
  drive mode/1 -> Mux/7  "veh2_drive_mode"
  max_accel/1 -> Mux/8  "veh2_max_accel"
  max_decel/1 -> Mux/9  "veh2_max_decel"
  max_spd/1 -> Mux/10  "veh2_max_spd"
  run_flag/1 -> Mux/11  "veh2_run_flag"
  comm_fault/1 -> Mux/12  "comm_pre_fault"
  pre_run_flag/1 -> Mux/13  "pre_run_flag"
  pre drive mode/1 -> Mux/14  "pre_drive_mode"
  lead drive mode/1 -> Mux/15  "lead_drive_mode"
  lead run flag/1 -> Mux/16  "lead_run_flag"
  lead a/1 -> Mux/17  "lead_a"
  lead v/1 -> Mux/18  "lead_v"
  d_to_lead_est/1 -> Mux/19  "rel_d_to_lead_est"
  des_d_gap_to_lead/1 -> Mux/20  "des_d_gap_to_lead"

== system CACC_system_struct/CACC Control Code 1/Coordination/Activation ==
  In1 : Inport
  Demux : Demux  Outputs=6
  tag scope: fvehicle_0=global, fvehicle_1=global, fvehicle_2=global, fvehicle_3=global, fvehicle_4=global, fvehicle_5=global
  wires:
  In1/1 -> Demux/1
  Demux/1 -> [fvehicle_0]
  Demux/2 -> [fvehicle_1]
  Demux/3 -> [fvehicle_2]
  Demux/4 -> [fvehicle_3]
  Demux/5 -> [fvehicle_4]
  Demux/6 -> [fvehicle_5]

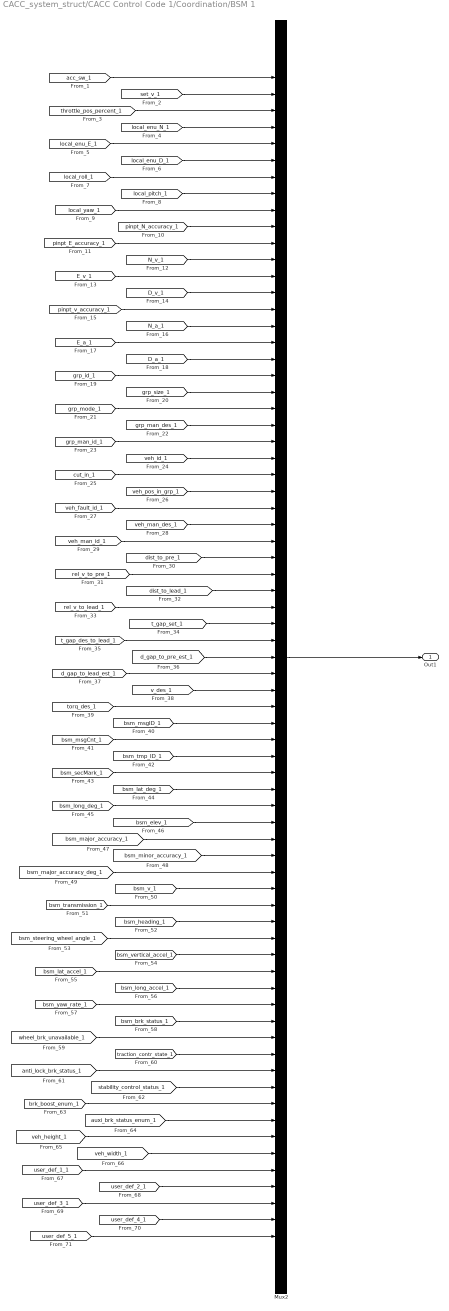
== system CACC_system_struct/CACC Control Code 1/Coordination/BSM 1 ==
  Mux2 : Mux  Inputs=71
  Out1 : Outport
  wires:
  Mux2/1 -> Out1/1
  [user_def_5_1] -> Mux2/71
  [user_def_4_1] -> Mux2/70
  [user_def_3_1] -> Mux2/69
  [user_def_2_1] -> Mux2/68
  [user_def_1_1] -> Mux2/67
  [brk_boost_enum_1] -> Mux2/63
  [auxi_brk_status_enum_1] -> Mux2/64
  [veh_width_1] -> Mux2/66
  [veh_height_1] -> Mux2/65
  [stability_control_status_1] -> Mux2/62
  [anti_lock_brk_status_1] -> Mux2/61
  [traction_contr_state_1] -> Mux2/60
  [wheel_brk_unavailable_1] -> Mux2/59
  [bsm_brk_status_1] -> Mux2/58
  [bsm_yaw_rate_1] -> Mux2/57
  [bsm_long_accel_1] -> Mux2/56
  [bsm_lat_accel_1] -> Mux2/55
  [bsm_vertical_accel_1] -> Mux2/54
  [bsm_steering_wheel_angle_1] -> Mux2/53
  [bsm_heading_1] -> Mux2/52
  [bsm_transmission_1] -> Mux2/51
  [bsm_v_1] -> Mux2/50
  [bsm_major_accuracy_deg_1] -> Mux2/49
  [bsm_minor_accuracy_1] -> Mux2/48
  [bsm_major_accuracy_1] -> Mux2/47
  [bsm_elev_1] -> Mux2/46
  [bsm_long_deg_1] -> Mux2/45
  [bsm_lat_deg_1] -> Mux2/44
  [bsm_secMark_1] -> Mux2/43
  [bsm_tmp_ID_1] -> Mux2/42
  [bsm_msgCnt_1] -> Mux2/41
  [bsm_msgID_1] -> Mux2/40
  [torq_des_1] -> Mux2/39
  [v_des_1] -> Mux2/38
  [d_gap_to_lead_est_1] -> Mux2/37
  [d_gap_to_pre_est_1] -> Mux2/36
  [t_gap_des_to_lead_1] -> Mux2/35
  [t_gap_set_1] -> Mux2/34
  [rel_v_to_lead_1] -> Mux2/33
  [dist_to_lead_1] -> Mux2/32
  [rel_v_to_pre_1] -> Mux2/31
  [dist_to_pre_1] -> Mux2/30
  [veh_man_id_1] -> Mux2/29
  [veh_man_des_1] -> Mux2/28
  [veh_fault_id_1] -> Mux2/27
  [veh_pos_in_grp_1] -> Mux2/26
  [acc_sw_1] -> Mux2/1
  [set_v_1] -> Mux2/2
  [throttle_pos_percent_1] -> Mux2/3
  [local_enu_N_1] -> Mux2/4
  [local_enu_E_1] -> Mux2/5
  [local_enu_D_1] -> Mux2/6
  [local_roll_1] -> Mux2/7
  [local_pitch_1] -> Mux2/8
  [local_yaw_1] -> Mux2/9
  [pinpt_N_accuracy_1] -> Mux2/10
  [pinpt_E_accuracy_1] -> Mux2/11
  [N_v_1] -> Mux2/12
  [E_v_1] -> Mux2/13
  [D_v_1] -> Mux2/14
  [pinpt_v_accuracy_1] -> Mux2/15
  [N_a_1] -> Mux2/16
  [E_a_1] -> Mux2/17
  [D_a_1] -> Mux2/18
  [grp_id_1] -> Mux2/19
  [grp_size_1] -> Mux2/20
  [grp_mode_1] -> Mux2/21
  [grp_man_des_1] -> Mux2/22
  [grp_man_id_1] -> Mux2/23
  [veh_id_1] -> Mux2/24
  [cut_in_1] -> Mux2/25
